simulink model "sampleModel1877"  (R2023a)
settings: Solver=VariableStepAuto  StartTime=0.0  StopTime=10.0  RelTol=1e-3
libraries: hdlsllib x8, simulink x2
settings Model: Creator=user1  LastModifiedBy=user1

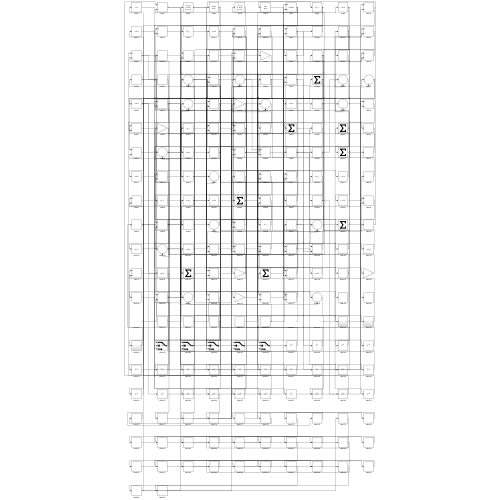
[thumbnail: Simulink's stored preview of the top-level diagram]
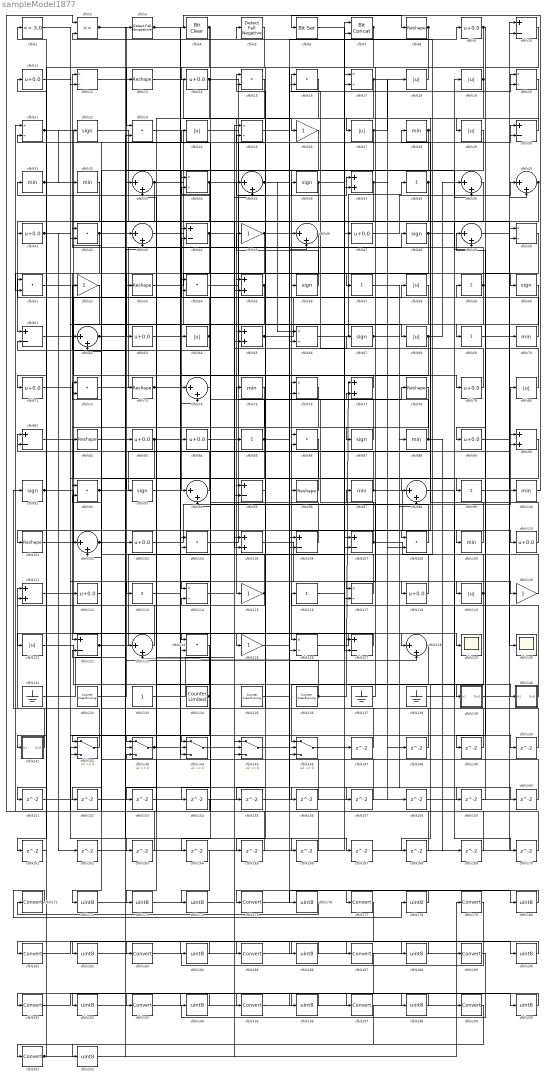
== system sampleModel1877 ==
  cfblk1 : hdlsllib/Logic and Bit Operations/Compare To Constant  relop=<=  const=3.0  OutDataTypeStr=boolean
  cfblk{10,30,44,61,81,95,106..107,122,127} (10 alike) : Sum  Inputs=+-
  cfblk{28,31..32,70,75,88,97,100,109} (9 alike) : MinMax
  cfblk{8,13,53,73,78,82,96,101} (8 alike) : Reshape
  cfblk{33,35,39..40,43,46,49,62,74,94,98,102,123,128} (14 alike) : Sum  Inputs=|++
  cfblk{9,11,14,41,47,63,71,79,83..84,89,103,110,112,118} (15 alike) : Bias  Bias=0.0  SaturateOnIntegerOverflow=off
  cfblk{15..16,23,42,51,54,72,86,92,104,108,124} (12 alike) : DotProduct  OutDataTypeStr=Inherit: Inherit via internal rule
  cfblk{37,55,65,77,90,105,111} (7 alike) : Sum
  cfblk{38,57,59,69,85,99,113,116} (8 alike) : Sum  Inputs=+
  cfblk{12,17,20..21,25,34,50,66,76,114,117,126} (12 alike) : Product  Inputs=*/  RndMeth=Zero  SaturateOnIntegerOverflow=on
  cfblk{26,45,52,115,120,125} (6 alike) : Gain
  cfblk{18..19,24,27,29,58,64,68,80,119,121} (11 alike) : Abs  SaturateOnIntegerOverflow=off
  cfblk129 : Scope
  cfblk130 : Scope
  cfblk131 : Ground
  cfblk132 : hdlsllib/Sources/Counter Free-Running  NumBits=16  tsamp=-1
  cfblk133 : Constant  SampleTime=-1
  cfblk134 : hdlsllib/Sources/Counter Limited  uplimit=7  tsamp=-1
  cfblk135 : hdlsllib/Sources/Counter Free-Running  NumBits=16  tsamp=-1
  cfblk136 : hdlsllib/Sources/Counter Free-Running  NumBits=16  tsamp=-1
  cfblk137 : Ground
  cfblk138 : Ground
  cfblk139 : Subsystem
      settings: LibrarySourceBlock=|
      | hdlsllib/Ports &
      | Subsystems/Subsystem
  cfblk140 : Subsystem
      settings: LibrarySourceBlock=|
      | hdlsllib/Ports &
      | Subsystems/Subsystem
  cfblk141 : Subsystem
      settings: LibrarySourceBlock=|
      | hdlsllib/Ports &
      | Subsystems/Subsystem
  cfblk{142..146} (5 alike) : Switch  SaturateOnIntegerOverflow=off  InputSameDT=off
  cfblk{147..170} (24 alike) : Delay  SampleTime=1
  cfblk{171,175,177,179,181,183,185,187,189,191,193,195,197,199,201} (15 alike) : DataTypeConversion  SaturateOnIntegerOverflow=off  RndMeth=Floor
  cfblk{172..174,176,178,180,182,184,186,188,190,192,194,196,198,200,202} (17 alike) : DataTypeConversion  OutDataTypeStr=uint8  SaturateOnIntegerOverflow=off  RndMeth=Floor
  cfblk2 : RelationalOperator  Operator=<=  OutDataTypeStr=boolean  InputSameDT=off
  cfblk{22,36,48,56,60,67,87,91,93} (9 alike) : Signum
  cfblk3 : hdlsllib/Logic and Bit Operations/Detect Fall Nonpositive  vinit=0  OutDataTypeStr=boolean
  cfblk4 : simulink/Logic and Bit Operations/Bit Clear  iBit=0
      settings: LibrarySourceBlock=|
      | hdlsllib/Logic and Bit
      | Operations/Bit Clear
  cfblk5 : hdlsllib/Logic and Bit Operations/Detect Fall Negative  vinit=0  OutDataTypeStr=boolean
  cfblk6 : simulink/Logic and Bit Operations/Bit Set  iBit=0
      settings: LibrarySourceBlock=|
      | hdlsllib/Logic and Bit
      | Operations/Bit Set
  cfblk7 : hdlsllib/Logic and Bit Operations/Bit Concat  numInputs=2
  wires:
  cfblk21/1 -> cfblk68/1, cfblk32/1
  cfblk28/1 -> cfblk101/1, cfblk106/2
  cfblk104/1 -> cfblk37/1
  cfblk142/1 -> cfblk91/1
  cfblk107/1 -> cfblk5/1, cfblk76/1
  cfblk87/1 -> cfblk31/1
  cfblk13/1 -> cfblk26/1
  cfblk132/1 -> cfblk3/1
  cfblk136/1 -> cfblk77/1, cfblk123/2
  cfblk46/1 -> cfblk122/1
  cfblk31/1 -> cfblk79/1, cfblk73/1
  cfblk29/1 -> cfblk94/1
  cfblk74/1 -> cfblk144/1
  cfblk5/1 -> cfblk23/1
  cfblk10/1 -> cfblk89/1
  cfblk15/1 -> cfblk115/1
  cfblk123/1 -> cfblk83/1
  cfblk53/1 -> cfblk60/1
  cfblk118/1 -> cfblk103/1
  cfblk66/1 -> cfblk38/1
  cfblk77/1 -> cfblk74/1
  cfblk141/1(Out1) -> cfblk111/1
  cfblk27/1 -> cfblk126/1, cfblk18/1
  cfblk68/1 -> cfblk86/1, cfblk39/1
  cfblk19/1 -> cfblk14/1, cfblk98/1, cfblk104/2
  cfblk103/1 -> cfblk80/1
  cfblk89/1 -> cfblk90/1
  cfblk105/1 -> cfblk118/1
  cfblk100/1 -> cfblk6/1
  cfblk59/1 -> cfblk12/1, cfblk164/1
  cfblk33/1 -> cfblk57/1, cfblk95/2, cfblk55/2, cfblk161/1
  cfblk122/1 -> cfblk17/1, cfblk24/1
  cfblk90/1 -> cfblk125/1
  cfblk96/1 -> cfblk43/1
  cfblk92/1 -> cfblk70/1, cfblk167/1
  cfblk54/1 -> cfblk36/1
  cfblk114/1 -> cfblk120/1
  cfblk115/1 -> cfblk111/2, cfblk54/1, cfblk21/2
  cfblk61/1 -> cfblk52/1
  cfblk4/1 -> cfblk12/2, cfblk84/1
  cfblk101/1 -> cfblk7/1
  cfblk88/1 -> cfblk75/1, cfblk169/1
  cfblk79/1 -> cfblk16/1
  cfblk143/1 -> cfblk64/1, cfblk33/2
  cfblk78/1 -> cfblk114/1
  cfblk32/1 -> cfblk61/1
  cfblk110/1 -> cfblk86/2
  cfblk135/1 -> cfblk16/2
  cfblk72/1 -> cfblk48/1
  cfblk139/1(Out1) -> cfblk50/1
  cfblk20/1 -> cfblk124/1
  cfblk82/1 -> cfblk139/1(In1)
  cfblk45/1 -> cfblk46/2, cfblk105/2
  cfblk49/1 -> cfblk100/1
  cfblk30/1 -> cfblk29/1
  cfblk84/1 -> cfblk78/1
  cfblk43/1 -> cfblk85/1
  cfblk6/1 -> cfblk47/1
  cfblk23/1 -> cfblk105/1
  cfblk127/1 -> cfblk121/1
  cfblk116/1 -> cfblk17/2
  cfblk38/1 -> cfblk41/1, cfblk126/2
  cfblk99/1 -> cfblk130/1
  cfblk14/1 -> cfblk107/1, cfblk144/3
  cfblk63/1 -> cfblk65/1
  cfblk52/1 -> cfblk92/1
  cfblk9/1 -> cfblk69/1, cfblk141/1(In1)
  cfblk62/1 -> cfblk9/1, cfblk99/1
  cfblk91/1 -> cfblk129/1, cfblk166/1
  cfblk35/1 -> cfblk50/2, cfblk66/1
  cfblk140/1(Out1) -> cfblk116/1
  cfblk25/1 -> cfblk110/1
  cfblk41/1 -> cfblk112/1, cfblk162/1, cfblk163/1
  cfblk121/1 -> cfblk140/1(In1)
  cfblk126/1 -> cfblk128/1
  cfblk22/1 -> cfblk124/2
  cfblk11/1 -> cfblk93/1
  cfblk106/1 -> cfblk62/1
  cfblk138/1 -> cfblk19/1
  cfblk67/1 -> cfblk88/1, cfblk98/2
  cfblk37/1 -> cfblk71/1, cfblk158/1
  cfblk80/1 -> cfblk59/1
  cfblk18/1 -> cfblk13/1
  cfblk85/1 -> cfblk33/1, cfblk159/1, cfblk173/1
  cfblk44/1 -> cfblk63/1, cfblk76/2
  cfblk94/1 -> cfblk81/1
  cfblk69/1 -> cfblk10/2
  cfblk119/1 -> cfblk15/1, cfblk168/1
  cfblk93/1 -> cfblk58/1
  cfblk3/1 -> cfblk8/1, cfblk96/1
  cfblk83/1 -> cfblk4/1, cfblk102/2, cfblk74/2
  cfblk128/1 -> cfblk146/1
  cfblk58/1 -> cfblk107/2
  cfblk7/1 -> cfblk2/2, cfblk127/2, cfblk66/2
  cfblk34/1 -> cfblk30/1, cfblk42/2
  cfblk137/1 -> cfblk97/1
  cfblk134/1 -> cfblk142/1, cfblk51/1, cfblk144/2
  cfblk48/1 -> cfblk56/1, cfblk20/1
  cfblk81/1 -> cfblk123/1
  cfblk36/1 -> cfblk108/1, cfblk151/1, cfblk152/1
  cfblk71/1 -> cfblk43/2
  cfblk120/1 -> cfblk72/1
  cfblk108/1 -> cfblk22/1
  cfblk109/1 -> cfblk28/1
  cfblk47/1 -> cfblk40/1
  cfblk113/1 -> cfblk104/1
  cfblk131/1 -> cfblk30/2
  cfblk17/1 -> cfblk27/1, cfblk148/1
  cfblk95/1 -> cfblk35/1
  cfblk125/1 -> cfblk77/2
  cfblk16/1 -> cfblk143/1
  cfblk65/1 -> cfblk7/2, cfblk20/2
  cfblk51/1 -> cfblk113/1
  cfblk117/1 -> cfblk53/1
  cfblk70/1 -> cfblk42/1
  cfblk133/1 -> cfblk35/2
  cfblk55/1 -> cfblk95/1, cfblk142/3
  cfblk56/1 -> cfblk45/1
  cfblk97/1 -> cfblk109/1, cfblk25/2, cfblk108/2
  cfblk42/1 -> cfblk51/2, cfblk156/1, cfblk157/1
  cfblk60/1 -> cfblk146/2
  cfblk40/1 -> cfblk87/1, cfblk54/2
  cfblk144/1 -> cfblk67/1
  cfblk64/1 -> cfblk44/2, cfblk61/2
  cfblk24/1 -> cfblk106/1
  cfblk8/1 -> cfblk55/1, cfblk117/1
  cfblk2/1 -> cfblk34/1, cfblk39/2
  cfblk1/1 -> cfblk49/2
  cfblk75/1 -> cfblk102/1
  cfblk12/1 -> cfblk146/3
  cfblk73/1 -> cfblk127/1, cfblk117/2
  cfblk102/1 -> cfblk128/2, cfblk119/1
  cfblk26/1 -> cfblk82/1
  cfblk146/1 -> cfblk147/1
  cfblk147/1 -> cfblk94/2
  cfblk148/1 -> cfblk72/2
  cfblk50/1 -> cfblk149/1
  cfblk149/1 -> cfblk114/2
  cfblk111/1 -> cfblk150/1
  cfblk150/1 -> cfblk15/2
  cfblk151/1 -> cfblk65/2
  cfblk152/1 -> cfblk62/2
  cfblk124/1 -> cfblk153/1
  cfblk153/1 -> cfblk46/1
  cfblk86/1 -> cfblk154/1
  cfblk154/1 -> cfblk2/1
  cfblk39/1 -> cfblk155/1
  cfblk155/1 -> cfblk90/2
  cfblk156/1 -> cfblk143/2
  cfblk157/1 -> cfblk92/2
  cfblk158/1 -> cfblk10/1
  cfblk159/1 -> cfblk49/1
  cfblk57/1 -> cfblk160/1
  cfblk160/1 -> cfblk44/1
  cfblk161/1 -> cfblk81/2
  cfblk162/1 -> cfblk37/2
  cfblk163/1 -> cfblk122/2
  cfblk76/1 -> cfblk165/1
  cfblk165/1 -> cfblk21/1
  cfblk166/1 -> cfblk142/2
  cfblk167/1 -> cfblk40/2
  cfblk168/1 -> cfblk143/3
  cfblk169/1 -> cfblk34/2
  cfblk98/1 -> cfblk170/1
  cfblk170/1 -> cfblk1/1
  cfblk112/1 -> cfblk172/1
  cfblk172/1 -> cfblk145/1
  cfblk173/1 -> cfblk145/2
  cfblk164/1 -> cfblk174/1
  cfblk174/1 -> cfblk145/3
  cfblk145/1 -> cfblk176/1
  cfblk176/1 -> cfblk171/1
  cfblk171/1 -> cfblk178/1
  cfblk178/1 -> cfblk175/1
  cfblk175/1 -> cfblk180/1
  cfblk180/1 -> cfblk177/1
  cfblk177/1 -> cfblk182/1
  cfblk182/1 -> cfblk179/1
  cfblk179/1 -> cfblk184/1
  cfblk184/1 -> cfblk181/1
  cfblk181/1 -> cfblk186/1
  cfblk186/1 -> cfblk183/1
  cfblk183/1 -> cfblk188/1
  cfblk188/1 -> cfblk185/1
  cfblk185/1 -> cfblk190/1
  cfblk190/1 -> cfblk187/1
  cfblk187/1 -> cfblk192/1
  cfblk192/1 -> cfblk189/1
  cfblk189/1 -> cfblk194/1
  cfblk194/1 -> cfblk191/1
  cfblk191/1 -> cfblk196/1
  cfblk196/1 -> cfblk193/1
  cfblk193/1 -> cfblk198/1
  cfblk198/1 -> cfblk195/1
  cfblk199/1 -> cfblk201/1
  cfblk195/1 -> cfblk200/1
  cfblk200/1 -> cfblk197/1
  cfblk201/1 -> cfblk23/2, cfblk25/1, cfblk11/1
  cfblk197/1 -> cfblk202/1
  cfblk202/1 -> cfblk199/1

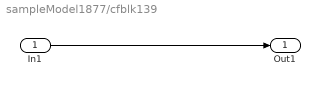
== system sampleModel1877/cfblk139 ==
  In1 : Inport
  Out1 : Outport
  wires:
  In1/1 -> Out1/1

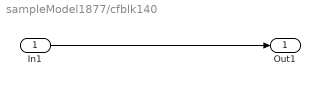
== system sampleModel1877/cfblk140 ==
  In1 : Inport
  Out1 : Outport
  wires:
  In1/1 -> Out1/1

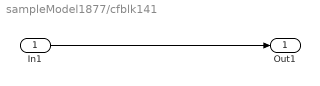
== system sampleModel1877/cfblk141 ==
  In1 : Inport
  Out1 : Outport
  wires:
  In1/1 -> Out1/1
